simulink model "SEMINAR_DFIG"  (R2014a)
settings: Solver=ode23tb  StartTime=0.0  StopTime=10.0  RelTol=1e-3
undefined symbols (not defined in the file or in its folder): o
libraries: powerlib x17, powerlib_meascontrol x7, simulink x4
settings Model: Creator=user  LastModifiedBy=ninad gaikawad

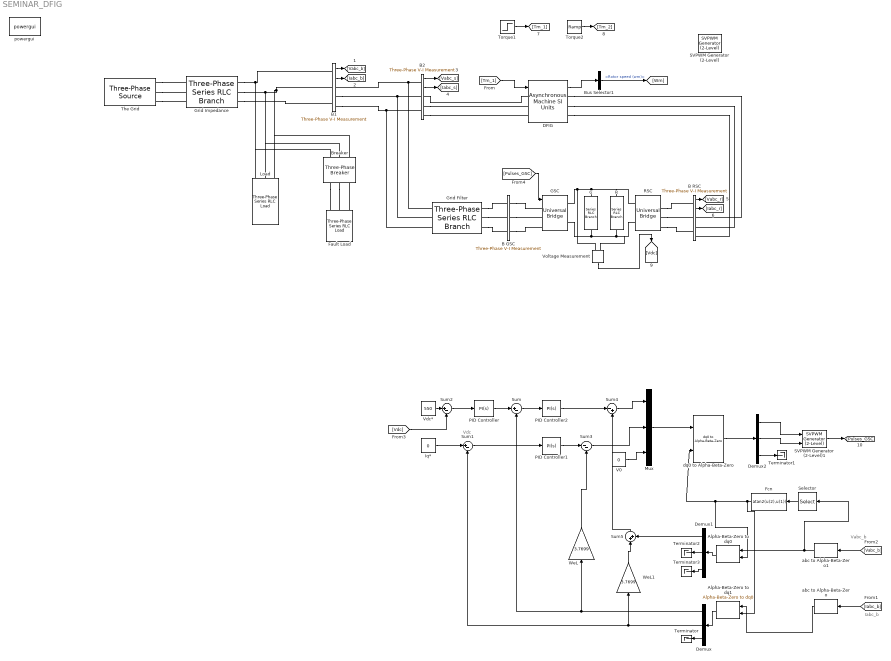
== system SEMINAR_DFIG ==
  note: Vdc
  note: Iabc_b
  note: Vabc_b
  Alpha-Beta-Zero to dq0 : powerlib_meascontrol/Transformations/Alpha-Beta-Zero to dq0  Alignment=Aligned with phase A axis
  Alpha-Beta-Zero to dq1 : powerlib_meascontrol/Transformations/Alpha-Beta-Zero to dq0  Alignment=Aligned with phase A axis
  B GSC : powerlib/Measurements/Three-Phase V-I Measurement  VoltageMeasurement=no  SetLabelV=off  LabelV=Vabc  Vpu=off  VpuLL=off  CurrentMeasurement=no  SetLabelI=off  LabelI=Iabc  Ipu=off  Pbase=100e6  Vbase=500e3  OutputType=Complex  PhasorSimulation=off  PSBequivalent=0
  B RSC : powerlib/Measurements/Three-Phase V-I Measurement  VoltageMeasurement=phase-to-ground  SetLabelV=off  LabelV=Vabc  Vpu=off  VpuLL=off  CurrentMeasurement=yes  SetLabelI=off  LabelI=Iabc  Ipu=off  Pbase=100e6  Vbase=500e3  OutputType=Complex  PhasorSimulation=off  PSBequivalent=0
  B1 : powerlib/Measurements/Three-Phase V-I Measurement  VoltageMeasurement=phase-to-ground  SetLabelV=off  LabelV=Vabc  Vpu=off  VpuLL=off  CurrentMeasurement=yes  SetLabelI=off  LabelI=Iabc  Ipu=off  Pbase=100e6  Vbase=500e3  OutputType=Complex  PhasorSimulation=off  PSBequivalent=0
  B2 : powerlib/Measurements/Three-Phase V-I Measurement  VoltageMeasurement=phase-to-ground  SetLabelV=off  LabelV=Vabc  Vpu=off  VpuLL=off  CurrentMeasurement=yes  SetLabelI=off  LabelI=Iabc  Ipu=off  Pbase=100e6  Vbase=500e3  OutputType=Complex  PhasorSimulation=off  PSBequivalent=0
  Breaker : powerlib/Elements/Three-Phase Breaker  InitialState=open  SwitchA=on  SwitchB=on  SwitchC=on  SwitchTimes="[1/60  5/60]"  External=off  BreakerResistance=0.01  SnubberResistance=1e6  SnubberCapacitance=inf  Measurements=None
  Bus Selector1 : BusSelector  OutputSignals=Mechanical.Rotor speed (wm)
  C : powerlib/Elements/Series RLC Branch  LConnTagsString=__new0  RConnTagsString=__new0  BranchType=C  Resistance=1  Inductance=1e-3  SetiL0=off  InitialCurrent=0  Capacitance=0.0024  Setx0=off  InitialVoltage=0  Measurements=None
  DFIG : powerlib/Machines/Asynchronous Machine SI Units  PresetModel=No  MechanicalLoad=Torque Tm  ShowDetailedParameters=on  RotorType=Wound  ReferenceFrame=Rotor  Units=SI  MeasurementBus=off  NominalParameters=[8e+03 415 50]  Stator=[1.06 0.2065]  Rotor=[0.80 0.0810]  Cage1=[ 0.022 0.226/377]  Cage2=[ 0.022 0.226/377]  Lm=0.02135  Mechanical=[0.4 0.06 3]  PolePairs=2  InitialConditions=[1 0 0 0 0 0 0 0]  SimulateSaturation=off  Saturation=[14.03593122, 27.81365428, 53.79336849, 72.68890987, 97.98006896, 148.6815601, 215.7428561, 302.9841135, 420.4778367 ; 230, 322, 414, 460, 506, 552, 598, 644, 690]  LoadFlowParameters=1492000  TsPowergui=0  TsBlock=-1  IterativeModel=Trapezoidal non iterative  Pmec=0
  Demux : Demux  Outputs=3
  Demux1 : Demux  Outputs=3
  Demux2 : Demux  Outputs=3
  Fault Load : powerlib/Elements/Three-Phase Series RLC Load  LConnTagsString=A|B|C  Configuration=Y (grounded)  NominalVoltage=1000  NominalFrequency=60  ActivePower=0.05e+3  InductivePower=0  CapacitivePower=0  Measurements=None  LoadType=constant Z
  Fcn : Fcn  Expr=atan2(u(2),u(1))
  GSC : powerlib/Power Electronics/Universal Bridge  Arms=3  SnubberResistance=1e5  SnubberCapacitance=inf  Device=IGBT / Diodes  Ron=1e-3  Lon=0  ForwardVoltages="[  0  0  ]"  ForwardVoltage=0  GTOparameters=[ 10e-6 , 20e-6 ]  IGBTparameters=[ 1e-6 , 2e-6 ]  Measurements=None  Measurements_2=None  converterType=Rectifier
  Grid Filter : powerlib/Elements/Three-Phase Series RLC Branch  LConnTagsString=A|B|C  RConnTagsString=A|B|C  BranchType=RL  Resistance=0.1  Inductance=0.012  Capacitance=1e-6  Measurements=None
  Grid Impedance : powerlib/Elements/Three-Phase Series RLC Branch  LConnTagsString=A|B|C  RConnTagsString=A|B|C  BranchType=RL  Resistance=1  Inductance=1e-3  Capacitance=1e-6  Measurements=None
  Iq* : Constant  Value=0
  Load : powerlib/Elements/Three-Phase Series RLC Load  LConnTagsString=A|B|C  Configuration=Y (grounded)  NominalVoltage=1000  NominalFrequency=50  ActivePower=5e+3  InductivePower=0  CapacitivePower=0  Measurements=None  LoadType=constant Z
  Mux : Mux  Inputs=3
  PID Controller : simulink/Continuous/PID Controller  Controller=PI  TimeDomain=Continuous-time  SampleTime=1  IntegratorMethod=Forward Euler  FilterMethod=Forward Euler  Form=Parallel  P=1  I=1  D=0  N=100  InitialConditionSource=internal  InitialConditionForIntegrator=0  InitialConditionForFilter=0  ExternalReset=none  LimitOutput=off  UpperSaturationLimit=inf  LowerSaturationLimit=-inf  LinearizeAsGain=on  AntiWindupMode=none  Kb=1  TrackingMode=off  Kt=1  PParamMin=[]  PParamMax=[]  IParamMin=[]  IParamMax=[]  DParamMin=[]  DParamMax=[]  NParamMin=[]  NParamMax=[]  KbParamMin=[]  KbParamMax=[]  KtParamMin=[]  KtParamMax=[]  POutMin=[]  POutMax=[]  IOutMin=[]  IOutMax=[]  DOutMin=[]  DOutMax=[]  NOutMin=[]  NOutMax=[]  KbOutMin=[]  KbOutMax=[]  KtOutMin=[]  KtOutMax=[]  IntegratorOutMin=[]  IntegratorOutMax=[]  FilterOutMin=[]  FilterOutMax=[]  SumOutMin=[]  SumOutMax=[]  SumI1OutMin=[]  SumI1OutMax=[]  SumI2OutMin=[]  SumI2OutMax=[]  SumI3OutMin=[]  SumI3OutMax=[]  SumDOutMin=[]  SumDOutMax=[]  SaturationOutMin=[]  SaturationOutMax=[]  IntegratorContinuousStateAttributes=''  IntegratorStateMustResolveToSignalObject=off  IntegratorRTWStateStorageClass=Auto  FilterContinuousStateAttributes=''  FilterStateMustResolveToSignalObject=off  FilterRTWStateStorageClass=Auto
  PID Controller1 : simulink/Continuous/PID Controller  Controller=PI  TimeDomain=Continuous-time  SampleTime=1  IntegratorMethod=Forward Euler  FilterMethod=Forward Euler  Form=Parallel  P=1  I=1  D=0  N=100  InitialConditionSource=internal  InitialConditionForIntegrator=0  InitialConditionForFilter=0  ExternalReset=none  LimitOutput=off  UpperSaturationLimit=inf  LowerSaturationLimit=-inf  LinearizeAsGain=on  AntiWindupMode=none  Kb=1  TrackingMode=off  Kt=1  PParamMin=[]  PParamMax=[]  IParamMin=[]  IParamMax=[]  DParamMin=[]  DParamMax=[]  NParamMin=[]  NParamMax=[]  KbParamMin=[]  KbParamMax=[]  KtParamMin=[]  KtParamMax=[]  POutMin=[]  POutMax=[]  IOutMin=[]  IOutMax=[]  DOutMin=[]  DOutMax=[]  NOutMin=[]  NOutMax=[]  KbOutMin=[]  KbOutMax=[]  KtOutMin=[]  KtOutMax=[]  IntegratorOutMin=[]  IntegratorOutMax=[]  FilterOutMin=[]  FilterOutMax=[]  SumOutMin=[]  SumOutMax=[]  SumI1OutMin=[]  SumI1OutMax=[]  SumI2OutMin=[]  SumI2OutMax=[]  SumI3OutMin=[]  SumI3OutMax=[]  SumDOutMin=[]  SumDOutMax=[]  SaturationOutMin=[]  SaturationOutMax=[]  IntegratorContinuousStateAttributes=''  IntegratorStateMustResolveToSignalObject=off  IntegratorRTWStateStorageClass=Auto  FilterContinuousStateAttributes=''  FilterStateMustResolveToSignalObject=off  FilterRTWStateStorageClass=Auto
  PID Controller2 : simulink/Continuous/PID Controller  Controller=PI  TimeDomain=Continuous-time  SampleTime=1  IntegratorMethod=Forward Euler  FilterMethod=Forward Euler  Form=Parallel  P=1  I=1  D=0  N=100  InitialConditionSource=internal  InitialConditionForIntegrator=0  InitialConditionForFilter=0  ExternalReset=none  LimitOutput=off  UpperSaturationLimit=inf  LowerSaturationLimit=-inf  LinearizeAsGain=on  AntiWindupMode=none  Kb=1  TrackingMode=off  Kt=1  PParamMin=[]  PParamMax=[]  IParamMin=[]  IParamMax=[]  DParamMin=[]  DParamMax=[]  NParamMin=[]  NParamMax=[]  KbParamMin=[]  KbParamMax=[]  KtParamMin=[]  KtParamMax=[]  POutMin=[]  POutMax=[]  IOutMin=[]  IOutMax=[]  DOutMin=[]  DOutMax=[]  NOutMin=[]  NOutMax=[]  KbOutMin=[]  KbOutMax=[]  KtOutMin=[]  KtOutMax=[]  IntegratorOutMin=[]  IntegratorOutMax=[]  FilterOutMin=[]  FilterOutMax=[]  SumOutMin=[]  SumOutMax=[]  SumI1OutMin=[]  SumI1OutMax=[]  SumI2OutMin=[]  SumI2OutMax=[]  SumI3OutMin=[]  SumI3OutMax=[]  SumDOutMin=[]  SumDOutMax=[]  SaturationOutMin=[]  SaturationOutMax=[]  IntegratorContinuousStateAttributes=''  IntegratorStateMustResolveToSignalObject=off  IntegratorRTWStateStorageClass=Auto  FilterContinuousStateAttributes=''  FilterStateMustResolveToSignalObject=off  FilterRTWStateStorageClass=Auto
  R : powerlib/Elements/Series RLC Branch  LConnTagsString=__new0  RConnTagsString=__new0  BranchType=R  Resistance=1  Inductance=1e-3  SetiL0=off  InitialCurrent=0  Capacitance=1e-6  Setx0=off  InitialVoltage=0  Measurements=None
  RSC : powerlib/Power Electronics/Universal Bridge  Arms=3  SnubberResistance=1e5  SnubberCapacitance=inf  Device=IGBT / Diodes  Ron=1e-3  Lon=0  ForwardVoltages="[  0  0  ]"  ForwardVoltage=0  GTOparameters=[ 10e-6 , 20e-6 ]  IGBTparameters=[ 1e-6 , 2e-6 ]  Measurements=None  Measurements_2=None  converterType=Rectifier
  SVPWM Generator (2-Level) : powerlib_meascontrol/Pulse & Signal Generators/SVPWM Generator (2-Level)  InputType=Magnitude-Angle (rad)  SwitchingPattern=Pattern #1  Fc=2000  ParUref=[0.8 -30 50]  Ts=0
  SVPWM Generator (2-Level)1 : powerlib_meascontrol/Pulse & Signal Generators/SVPWM Generator (2-Level)  InputType=alpha-beta components  SwitchingPattern=Pattern #1  Fc=27*50  ParUref=[0.8 -30 50]  Ts=0
  Selector : Selector  InputPortWidth=3  Indices=[1 2]
  Sum : Sum  Inputs=|+-
  Sum1 : Sum  Inputs=|+-
  Sum2 : Sum  Inputs=|+-
  Sum3 : Sum  Inputs=|--
  Sum4 : Sum  Inputs=|-+
  Sum5 : Sum  Inputs=|++
  Terminator{,1..3} (4 alike) : Terminator
  The Grid : powerlib/Electrical Sources/Three-Phase Source  Voltage=415  PhaseAngle=0  Frequency=50  InternalConnection=Yg  SpecifyImpedance=off  Resistance=0.8929  Inductance=o  ShortCircuitLevel=100e6  BaseVoltage=25e3  XRratio=7  BusType=swing  Pref=0  Qref=0  Qmin=-inf  Qmax=inf
  Torque1 : Step  Time=-1  SampleTime=0
  Torque2 : simulink/Sources/Ramp  slope=-1  start=0  X0=0
  V0 : Constant  Value=0
  Vdc* : Constant  Value=550
  Voltage Measurement : powerlib/Measurements/Voltage Measurement  PhasorSimulation=off  OutputType=Complex  PSBequivalent=0
  WeL : Gain  Gain=3.7699
  WeL1 : Gain  Gain=3.7699
  abc to Alpha-Beta-Zero : powerlib_meascontrol/Transformations/abc to Alpha-Beta-Zero
  abc to Alpha-Beta-Zero1 : powerlib_meascontrol/Transformations/abc to Alpha-Beta-Zero
  dq0 to Alpha-Beta-Zero : powerlib_meascontrol/Transformations/dq0 to Alpha-Beta-Zero  Alignment=90 degrees behind phase A axis
  powergui : powerlib/powergui  Priority=1  SimulationMode=Continuous  SolverType=Tustin  SampleTime=50e-6  frequency=60  SPID=off  DisableSnubberDevices=off  DisableRonSwitches=off  DisableVfSwitches=off  SwTol=0  Interpol=off  DisplayEquations=off  Ts=0  methode=off  frequencyindice=60  Pbase=100e6  ErrMax=1e-4  Iterations=50  UnitsV=kV  UnitsW=MW  FunctionMessages=off  echomessages=off  HookPort=off  EnableUseOfTLC=off  x0status=blocks  RestoreLinks=warning  ResistiveCurrentMeasurement=off  Frange=[0:2:500]  Ylog=off  Xlog=on  ShowGrid=off  save=off  variable=ZData  structure=0  ZoomFFT=off  StartTime=0.0  cycles=1  DisplayStyle=1  fundamental=60  FreqAxis=off  MaxFrequency=1000  frequencyindicesteady=1  RmsSteady=1  display=off
  wires:
  DFIG/1 -> Bus Selector1/1
  Bus Selector1/1 -> [Wm]  "<Rotor speed (wm)>"
  B1/1 -> [Vabc_b]
  B1/2 -> [Iabc_b]
  B2/1 -> [Vabc_s]
  B2/2 -> [Iabc_s]
  B RSC/1 -> [Vabc_r]
  B RSC/2 -> [Iabc_r]
  Torque1/1 -> [Tm_1]
  Torque2/1 -> [Tm_2]
  [Tm_1] -> DFIG/1
  Voltage Measurement/1 -> [Vdc]
  Demux1/3 -> Terminator3/1
  Demux/3 -> Terminator/1
  Alpha-Beta-Zero to dq1/1 -> Demux/1
  Fcn/1 -> Alpha-Beta-Zero to dq1/2, dq0 to Alpha-Beta-Zero/2, Alpha-Beta-Zero to dq0/2
  abc to Alpha-Beta-Zero1/1 -> Selector/1, Alpha-Beta-Zero to dq0/1
  abc to Alpha-Beta-Zero/1 -> Alpha-Beta-Zero to dq1/1
  Alpha-Beta-Zero to dq0/1 -> Demux1/1
  [Vabc_b] -> abc to Alpha-Beta-Zero1/1
  Demux1/2 -> Terminator2/1
  [Iabc_b] -> abc to Alpha-Beta-Zero/1
  Selector/1 -> Fcn/1
  Demux2/3 -> Terminator1/1
  Demux2/2 -> SVPWM Generator (2-Level)1/2
  Demux2/1 -> SVPWM Generator (2-Level)1/1
  dq0 to Alpha-Beta-Zero/1 -> Demux2/1
  Mux/1 -> dq0 to Alpha-Beta-Zero/1
  Sum4/1 -> Mux/1
  PID Controller1/1 -> Sum3/1
  Demux/1 -> WeL/1, Sum/2
  Demux1/1 -> Sum5/2
  PID Controller2/1 -> Sum4/1
  Demux/2 -> WeL1/1, Sum1/2
  Sum1/1 -> PID Controller1/1
  Sum5/1 -> Sum4/2
  Sum3/1 -> Mux/2
  WeL1/1 -> Sum5/1
  PID Controller/1 -> Sum/1
  Iq*/1 -> Sum1/1
  WeL/1 -> Sum3/2
  Sum2/1 -> PID Controller/1
  Vdc*/1 -> Sum2/1
  V0/1 -> Mux/3
  Sum/1 -> PID Controller2/1
  [Vdc] -> Sum2/2
  SVPWM Generator (2-Level)1/1 -> [Pulses_GSC]
  [Pulses_GSC] -> GSC/1
  connections:
  GSC/RConn1 -- RSC/RConn1 -- R/LConn1 -- C/LConn1 -- Voltage Measurement/LConn1
  GSC/RConn2 -- Voltage Measurement/LConn2 -- RSC/RConn2 -- R/RConn1 -- C/RConn1
  The Grid/RConn1 -- Grid Impedance/LConn1
  The Grid/RConn2 -- Grid Impedance/LConn2
  The Grid/RConn3 -- Grid Impedance/LConn3
  Breaker/RConn1 -- Fault Load/LConn1
  Breaker/RConn2 -- Fault Load/LConn2
  Grid Impedance/RConn2 -- Breaker/LConn2 -- Load/LConn2 -- Breaker/LConn3 -- Load/LConn3 -- B1/LConn2
  Grid Impedance/RConn3 -- B1/LConn3
  B1/RConn2 -- Grid Filter/LConn2 -- B2/LConn2
  B1/RConn3 -- Grid Filter/LConn3 -- B2/LConn3
  B2/LConn1 -- Grid Filter/LConn1 -- B1/RConn1
  Grid Impedance/RConn1 -- Breaker/LConn1 -- Load/LConn1 -- B1/LConn1
  Fault Load/LConn3 -- Breaker/RConn3
  B2/RConn1 -- DFIG/LConn1
  B2/RConn2 -- DFIG/LConn2
  B2/RConn3 -- DFIG/LConn3
  Grid Filter/RConn1 -- B GSC/LConn1
  Grid Filter/RConn2 -- B GSC/LConn2
  Grid Filter/RConn3 -- B GSC/LConn3
  B GSC/RConn3 -- GSC/LConn3
  B GSC/RConn2 -- GSC/LConn2
  B GSC/RConn1 -- GSC/LConn1
  RSC/LConn1 -- B RSC/LConn1
  RSC/LConn2 -- B RSC/LConn2
  RSC/LConn3 -- B RSC/LConn3
  DFIG/RConn1 -- B RSC/RConn1
  DFIG/RConn2 -- B RSC/RConn2
  DFIG/RConn3 -- B RSC/RConn3
